simulink model "Apontamento"  (R2024a)
settings: Solver=FixedStepAuto  StartTime=0.0  StopTime=tf  FixedStep=step_modelo  RelTol=1e-3
undefined symbols (not defined in the file or in its folder): man
settings Model: PauseTimes=1138  Creator=rodri  LastModifiedBy=rodri
settings RTWCC: GPUComputeCapability=3.5

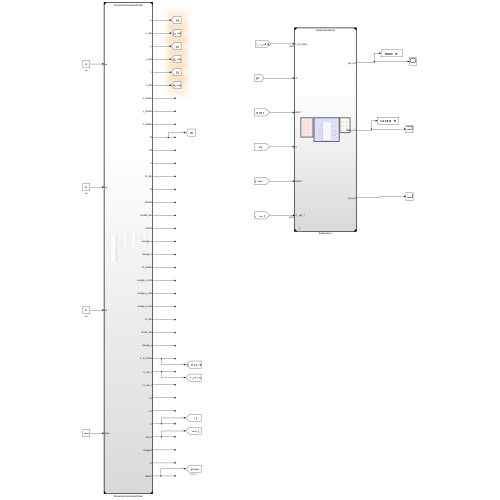
[thumbnail: Simulink's stored preview of the top-level diagram]
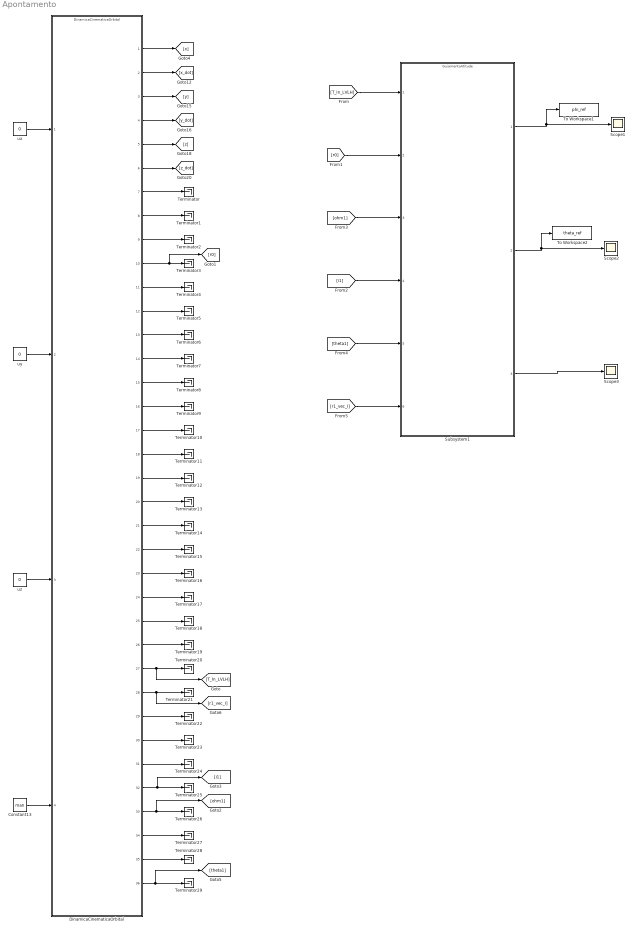
== system Apontamento ==
  Constant13 : Constant  Value=man  OutDataTypeStr=boolean
  DinamicaCinematicaOrbital : ModelReference  ModelNameDialog=DinamicaCinematicaOrbital  ModelReferenceVersion=5.0
  Scope1 : Scope
  Scope2 : Scope
  Scope3 : Scope
  Subsystem1 : ModelReference  ModelNameDialog=GuiamentoAtitude  ModelReferenceVersion=3.3
  Terminator{,1..29} (30 alike) : Terminator
  To Workspace1 : ToWorkspace  VariableName=phi_ref  SaveFormat=Timeseries  SampleTime=-1
  To Workspace2 : ToWorkspace  VariableName=theta_ref  SaveFormat=Timeseries  SampleTime=-1
  ux : Constant  Value=0
  uy : Constant  Value=0
  uz : Constant  Value=0
  wires:
  Subsystem1/1 -> To Workspace1/1, Scope1/1
  Subsystem1/2 -> Scope2/1, To Workspace2/1
  Subsystem1/3 -> Scope3/1
  DinamicaCinematicaOrbital/12 -> Terminator5/1
  DinamicaCinematicaOrbital/8 -> Terminator1/1
  uz/1 -> DinamicaCinematicaOrbital/3
  DinamicaCinematicaOrbital/6 -> [z_dot]
  DinamicaCinematicaOrbital/3 -> [y]
  DinamicaCinematicaOrbital/5 -> [z]
  DinamicaCinematicaOrbital/1 -> [x]
  DinamicaCinematicaOrbital/36 -> [theta1], Terminator29/1
  DinamicaCinematicaOrbital/13 -> Terminator6/1
  DinamicaCinematicaOrbital/25 -> Terminator18/1
  DinamicaCinematicaOrbital/34 -> Terminator27/1
  DinamicaCinematicaOrbital/19 -> Terminator12/1
  DinamicaCinematicaOrbital/15 -> Terminator8/1
  DinamicaCinematicaOrbital/30 -> Terminator23/1
  Constant13/1 -> DinamicaCinematicaOrbital/4
  DinamicaCinematicaOrbital/32 -> Terminator25/1, [i1]
  DinamicaCinematicaOrbital/9 -> Terminator2/1
  DinamicaCinematicaOrbital/2 -> [x_dot]
  DinamicaCinematicaOrbital/31 -> Terminator24/1
  DinamicaCinematicaOrbital/28 -> [r1_vec_I], Terminator21/1
  DinamicaCinematicaOrbital/27 -> [T_In_LVLH], Terminator20/1
  DinamicaCinematicaOrbital/11 -> Terminator4/1
  uy/1 -> DinamicaCinematicaOrbital/2
  DinamicaCinematicaOrbital/24 -> Terminator17/1
  DinamicaCinematicaOrbital/17 -> Terminator10/1
  DinamicaCinematicaOrbital/16 -> Terminator9/1
  DinamicaCinematicaOrbital/33 -> [ohm1], Terminator26/1
  ux/1 -> DinamicaCinematicaOrbital/1
  DinamicaCinematicaOrbital/35 -> Terminator28/1
  DinamicaCinematicaOrbital/29 -> Terminator22/1
  DinamicaCinematicaOrbital/18 -> Terminator11/1
  DinamicaCinematicaOrbital/21 -> Terminator14/1
  DinamicaCinematicaOrbital/23 -> Terminator16/1
  DinamicaCinematicaOrbital/7 -> Terminator/1
  DinamicaCinematicaOrbital/22 -> Terminator15/1
  DinamicaCinematicaOrbital/20 -> Terminator13/1
  DinamicaCinematicaOrbital/14 -> Terminator7/1
  DinamicaCinematicaOrbital/10 -> [r0], Terminator3/1
  DinamicaCinematicaOrbital/26 -> Terminator19/1
  DinamicaCinematicaOrbital/4 -> [y_dot]
  [T_In_LVLH] -> Subsystem1/1
  [r0] -> Subsystem1/2
  [ohm1] -> Subsystem1/3
  [i1] -> Subsystem1/4
  [theta1] -> Subsystem1/5
  [r1_vec_I] -> Subsystem1/6
